simulink model "gnc"  (R2025b)
settings: Solver=ode2  StartTime=0.0  StopTime=inf  FixedStep=1/100  RelTol=1e-3
PreLoadFcn:
  | gnc_PreLoadFcn
undefined symbols (not defined in the file or in its folder): DiscIntNeverNeededParam, dspblkCoreblockFVToolHelper, gcbh
libraries: simulink_extras x7, simulink x5, eeGeneralControl x5
(part 2 of 4)

== system gnc/INDI/Monitor ==
  note: uint64 timestamp
      | float32[3] track_cmd
      | float32[3] track_m
      | float32[3] track_err
      | float32[3] gamma_dot_pid
      | float32[2] chi_dot_pd
      | float32[3] track_dot_cmd
      | float32[3] track_dot_m
      | float32[3] track_dot_err
      | float32[3] att_inc_cmd
      | float32[5] att_cmd
      | float32[5] att_m
      | float32[5] att_err
      | float32[5] att_dot_cmd
      | float32 delta_t
      | float32 t_m
      | float32 t_c
      | float32 chi_dot_cmd
      | float32 chi_dot_m
      | float32 chi_dot_err
      | float32 chi_ddot_cmd
      | float32[3] pqr_cmd
      | float32[3] pqr_m
      | float32[3] pqr_err
      | float32[3] pqr_dot_cmd
      | float32[3] pqr_dot_m
      | float32[3] pqr_dot_err
      | float32[3] delta_act
      | float32[3] act_m
      | float32[3] act_c
      | float32 nw_c
  note: float32[3] track_cmd
      | float32[3] track_m
      | float32[3] track_err
      | float32[3] gamma_dot_pid
      | float32[2] chi_dot_pd
      | float32[3] track_dot_cmd
      | float32[3] track_dot_m
      | float32[3] track_dot_err
      | float32[3] att_inc_cmd
  note: float32[5] att_cmd
      | float32[5] att_m
      | float32[5] att_err
      | float32[5] att_dot_cmd
  note: float32 delta_t
      | float32 t_m
      | float32 t_c
  note: float32 chi_dot_cmd
      | float32 chi_dot_m
      | float32 chi_dot_err
      | float32 chi_ddot_cmd
      | float32[3] pqr_cmd
      | float32[3] pqr_m
      | float32[3] pqr_err
      | float32[3] pqr_dot_cmd
      | float32[3] pqr_dot_m
      | float32[3] pqr_dot_err
      | float32[3] delta_act
      | float32[3] act_m
      | float32[3] act_c
      | float32 nw_c
  rte_moni : Inport  OutDataTypeStr=single  PortDimensions=32
  att_moni : Inport  Port=2  OutDataTypeStr=single  PortDimensions=20
  thr_moni : Inport  Port=3  OutDataTypeStr=single  PortDimensions=3
  path_moni : Inport  Port=4  OutDataTypeStr=single  PortDimensions=26
  Bus Creator1 : BusCreator  Inputs=31  OutDataTypeStr=Bus: indi_monitor_bus
      settings: InheritFromInputs=off
  Bus Selector1 : BusSelector  OutputSignals=signal1,signal2,signal3,signal4
  Bus Selector2 : BusSelector  OutputSignals=signal1.signal1,signal1.signal2,signal1.signal3,signal1.signal4,signal1.signal5,signal1.signal6,signal1.signal7,signal1.signal8,signal1.signal9,signal1.signal10,signal2.signal1,signal2.signal2,signal2.signal3,signal3
  Bus Selector3 : BusSelector  OutputSignals=signal1.signal1,signal1.signal2,signal1.signal3,signal1.signal4,signal1.signal5,signal1.signal6,signal1.signal7,signal1.signal8,att_inc_reciprocal
  Constant : Constant  OutDataTypeStr=boolean
  Demux4 : Demux  Outputs=3
  indi_monitor : Outport  OutDataTypeStr=Bus: indi_monitor_bus
  wires:
  thr_moni/1 -> Demux4/1
  Constant/1 -> Bus Creator1/1  "valid"
  Bus Creator1/1 -> indi_monitor/1
  Demux4/1 -> Bus Creator1/15
  Demux4/2 -> Bus Creator1/16
  Demux4/3 -> Bus Creator1/17
  Bus Selector2/1 -> Bus Creator1/18  "<signal1>"
  Bus Selector2/2 -> Bus Creator1/19  "<signal2>"
  Bus Selector2/3 -> Bus Creator1/20  "<signal3>"
  Bus Selector2/4 -> Bus Creator1/21  "<signal4>"
  Bus Selector2/5 -> Bus Creator1/22  "<signal5>"
  Bus Selector2/6 -> Bus Creator1/23  "<signal6>"
  Bus Selector2/8 -> Bus Creator1/25  "<signal8>"
  Bus Selector2/9 -> Bus Creator1/26  "<signal9>"
  Bus Selector2/10 -> Bus Creator1/27  "<signal10>"
  Bus Selector2/7 -> Bus Creator1/24  "<signal7>"
  Bus Selector2/14 -> Bus Creator1/31  "<signal3>"
  Bus Selector2/13 -> Bus Creator1/30  "<signal3>"
  Bus Selector2/11 -> Bus Creator1/28  "<signal1>"
  Bus Selector2/12 -> Bus Creator1/29  "<signal2>"
  Bus Selector3/1 -> Bus Creator1/2  "<signal1>"
  Bus Selector3/2 -> Bus Creator1/3  "<signal2>"
  Bus Selector3/3 -> Bus Creator1/4  "<signal3>"
  Bus Selector3/4 -> Bus Creator1/5  "<signal4>"
  Bus Selector3/5 -> Bus Creator1/6  "<signal5>"
  Bus Selector3/6 -> Bus Creator1/7  "<signal6>"
  Bus Selector3/7 -> Bus Creator1/8  "<signal7>"
  Bus Selector3/8 -> Bus Creator1/9  "<signal8>"
  Bus Selector1/1 -> Bus Creator1/11  "<signal1>"
  Bus Selector1/2 -> Bus Creator1/12  "<signal2>"
  Bus Selector1/3 -> Bus Creator1/13  "<signal3>"
  Bus Selector1/4 -> Bus Creator1/14  "<signal4>"
  path_moni/1 -> Bus Selector3/1
  att_moni/1 -> Bus Selector1/1
  rte_moni/1 -> Bus Selector2/1
  Bus Selector3/9 -> Bus Creator1/10  "<att_inc_reciprocal>"

== system gnc/INDI/Path ==
  note: [alpha,theta,beta,psi,mu]
  note: for attitude dynamics
  note: float32[3] track_cmd
      | float32[3] track_m
      | float32[3] track_err
      | float32[3] gamma_dot_pid
      | float32[2] chi_dot_pd
      | float32[3] track_dot_cmd
      | float32[3] track_dot_m
      | float32[3] track_dot_err
      | float32[3] att_inc_cmd
  gachiv_c : Inport  OutDataTypeStr=single  PortDimensions=3
  acc_k : Inport  Port=2
  Vk : Inport  Port=3  OutDataTypeStr=single  PortDimensions=1
  att_m : Inport  Port=4
  gachi_m : Inport  Port=5  OutDataTypeStr=single  PortDimensions=2
  track_deriv : Inport  Port=6
  params : Inport  Port=7  OutDataTypeStr=Bus: gnc_parameterBus
  q_dyn : Inport  Port=8
  Bus Creator : BusCreator  Inputs=2
  Incremental_inversion : Subsystem
  MATLAB Function : MATLAB Function  TreatAsAtomicUnit=on
  Mux1 : Mux  Inputs=2
  Mux3 : Mux  Inputs=2
  Pseudo-control : Subsystem
  Selector1 : Selector  InputPortWidth=5  IndexOptions=Index vector (dialog)  Indices=[1 3 5]  OutputSizes=1
  Selector2 : Selector  InputPortWidth=3  IndexOptions=Index vector (dialog)  Indices=3  OutputSizes=1
  Selector3 : Selector  InputPortWidth=5  IndexOptions=Index vector (dialog)  Indices=5  OutputSizes=1
  d/dt_gachiv_m : Outport  OutDataTypeStr=single  PortDimensions=3
  angles_c : Outport  Port=2  OutDataTypeStr=single  PortDimensions=5
  path_moni : Outport  Port=3
  thr_inc : Outport  Port=4  OutDataTypeStr=single  PortDimensions=1
  wires:
  Incremental_inversion/1(angles_c) -> angles_c/1
  att_m/1 -> Selector3/1, Selector1/1
  acc_k/1 -> MATLAB Function/1(acc_k)
  Pseudo-control/2(d/dt_gachiv_e) -> Incremental_inversion/1(d/dt_gachiv_e)
  Mux1/1 -> Incremental_inversion/3(gachiv_m), Pseudo-control/5(gachiv_m)
  gachi_m/1 -> Mux1/1
  Vk/1 -> Mux1/2, MATLAB Function/2(Vk)
  Selector1/1 -> Incremental_inversion/4(abmu_m)
  Selector3/1 -> Pseudo-control/4(phi_m)
  MATLAB Function/2(v_dot) -> Mux3/2
  Mux3/1 -> Pseudo-control/1(d/dt_gachiv_m), d/dt_gachiv_m/1
  params/1 -> Incremental_inversion/2(params), Pseudo-control/3(para)
  Incremental_inversion/2(inc_cmd) -> Bus Creator/2, Selector2/1
  q_dyn/1 -> Incremental_inversion/5(q_dyn)
  Pseudo-control/1(path_moni) -> Bus Creator/1
  track_deriv/1 -> Mux3/1
  Bus Creator/1 -> path_moni/1
  Selector2/1 -> thr_inc/1
  gachiv_c/1 -> Pseudo-control/2(gachiv_c)

== system gnc/INDI/Rates to surfaces&brakes ==
  note: float32 chi_dot_cmd
      | float32 chi_dot_m
      | float32 chi_dot_err
      | float32 chi_ddot_cmd
      | float32[3] pqr_cmd
      | float32[3] pqr_m
      | float32[3] pqr_err
      | float32[3] pqr_dot_cmd
      | float32[3] pqr_dot_m
      | float32[3] pqr_dot_err
      | float32[3] delta_act
      | float32[3] act_m
      | float32[3] act_c
      | float32 nw
  q_dyn : Inport
  rate_m : Inport  Port=2
  rate_ctrl : Inport  Port=3
  act_m : Inport  Port=4  OutDataTypeStr=single  PortDimensions=4
  params : Inport  Port=5  OutDataTypeStr=Bus: gnc_parameterBus
  inc_margins : Inport  Port=6  OutDataTypeStr=single  PortDimensions=[3,2]
  act_limits : Inport  Port=7
  imu_filter : Inport  Port=8
  Bus Creator : BusCreator  Inputs=3
  Constant : Constant  Value=0  OutDataTypeStr=single
  Demux : Demux  Outputs=3
  Diff and Filter IMU : Subsystem
      settings: PortSchema="{\"entries\":[{\"content\":{\"sides\":[{\"content\":{\"connectorIds\":[\"In1\",\"In2\",\"In3\"]},\"type\":\"ConnectorPlacement.EquallySpacedRectSide\",\"uuid\":\"595f2c85-6cd2-4ac4-94a6-147e3cdaf62c\"},{\"content\":{\"connectorIds\":[\"Out1\",\"Out2\"],\"side\":\"RIGHT\"},\"type\":\"ConnectorPlacement.EquallySpacedRectSide\",\"uuid\":\"fac480cf-7efe-4f97-8544-e0f640d96e89\"},{\"content\":{\"connectorIds\":[\"In4\"],\"side\":\"TOP\"},\"type\":\"ConnectorPlacement.EquallySpacedRectSide\",\"uuid\":\"db60b5ab-e407-476e-aa28-a63f2500fd6d\"}]},\"type\":\"ConnectorPlacement.EquallySpacedConnector\",\"uuid\":\"42848a63-649d-42c6-8a03-05f224ad5118\"}],\"packageUris\":[\"http://schema.mathworks.com/mf0/Connector/R2020b\"],\"version\":\"1.0\"}"
  Incremental_inversion : Subsystem
      settings: PortSchema="{\"entries\":[{\"content\":{\"sides\":[{\"content\":{\"connectorIds\":[\"In1\",\"In2\",\"In3\",\"In4\",\"In5\"]},\"type\":\"ConnectorPlacement.EquallySpacedRectSide\",\"uuid\":\"2477ed7f-2e4a-4d34-9191-aa6cd1598ace\"},{\"content\":{\"connectorIds\":[\"Out1\",\"Out2\",\"Out3\"],\"side\":\"RIGHT\"},\"type\":\"ConnectorPlacement.EquallySpacedRectSide\",\"uuid\":\"a67f6923-e928-4938-ab2a-8a1d443bfb45\"},{\"content\":{\"connectorIds\":[\"In6\"],\"side\":\"TOP\"},\"type\":\"ConnectorPlacement.EquallySpacedRectSide\",\"uuid\":\"ece43f97-e3a7-408a-af02-d9e4d3d20b00\"}]},\"type\":\"ConnectorPlacement.EquallySpacedConnector\",\"uuid\":\"8ca6f7dd-4284-4525-a7ce-c1aaa2c7f949\"}],\"packageUris\":[\"http://schema.mathworks.com/mf0/Connector/R2020b\"],\"version\":\"1.0\"}"
  Pseudo-control : Subsystem
      settings: PortSchema="{\"entries\":[{\"content\":{\"sides\":[{\"content\":{\"connectorIds\":[\"In1\",\"In2\",\"In3\"]},\"type\":\"ConnectorPlacement.EquallySpacedRectSide\",\"uuid\":\"2477ed7f-2e4a-4d34-9191-aa6cd1598ace\"},{\"content\":{\"connectorIds\":[\"Out1\",\"Out2\"],\"side\":\"RIGHT\"},\"type\":\"ConnectorPlacement.EquallySpacedRectSide\",\"uuid\":\"a67f6923-e928-4938-ab2a-8a1d443bfb45\"},{\"content\":{\"connectorIds\":[\"In4\"],\"side\":\"TOP\"},\"type\":\"ConnectorPlacement.EquallySpacedRectSide\",\"uuid\":\"ece43f97-e3a7-408a-af02-d9e4d3d20b00\"}]},\"type\":\"ConnectorPlacement.EquallySpacedConnector\",\"uuid\":\"8ca6f7dd-4284-4525-a7ce-c1aaa2c7f949\"}],\"packageUris\":[\"http://schema.mathworks.com/mf0/Connector/R2020b\"],\"version\":\"1.0\"}"
  Scope : Scope  NumInputPorts=3
      settings: ActiveDisplayYMinimum=-0.13287401574803148  ActiveDisplayYMaximum=0.13779527559055116  DataLoggingVariableName=ScopeData6
  control_surfaces : Outport  OutDataTypeStr=single  PortDimensions=3
  rte_moni : Outport  Port=2  OutDataTypeStr=single  PortDimensions=32
  inc_moni : Outport  Port=3
  wires:
  Incremental_inversion/1(act) -> control_surfaces/1, Demux/1
  Incremental_inversion/3(srfc_moni) -> Bus Creator/2
  Pseudo-control/2(rte_moni) -> Bus Creator/1
  params/1 -> Diff and Filter IMU/4(params), Pseudo-control/4(param), Incremental_inversion/6(params)
  rate_m/1 -> Diff and Filter IMU/3(rates), Pseudo-control/2(rate_m)
  Pseudo-control/1(d/dt_pqr_e) -> Incremental_inversion/5(d/dt_pqr_e)
  act_m/1 -> Diff and Filter IMU/2(act_m)
  Incremental_inversion/2(inc_moni) -> inc_moni/1
  Diff and Filter IMU/2(d/dt_pqr_m) -> Pseudo-control/1(pqr_dot_m)
  Bus Creator/1 -> rte_moni/1
  Demux/2 -> Scope/2  "ele_cmd"
  Demux/3 -> Scope/3  "rud_cmd"
  Demux/1 -> Scope/1  "ail_cmd"
  Diff and Filter IMU/1(act_del) -> Incremental_inversion/4(act_del)
  q_dyn/1 -> Incremental_inversion/3(q_dyn)
  inc_margins/1 -> Incremental_inversion/2(inc_margins)
  act_limits/1 -> Incremental_inversion/1(act_limits)
  imu_filter/1 -> Diff and Filter IMU/1(imu_filter)
  Constant/1 -> Bus Creator/3
  rate_ctrl/1 -> Pseudo-control/3(rte_c)

== system gnc/INDI/Thrust ==
  note: float32 delta_t
      | float32 t_m
      | float32 t_c
  note: Current thrust
      | lever in [-1,1]
  note: Incremental thrust
      | command in [-1,1]
  note: Total thrust
      | command in [0,1]
  thr_inc : Inport  OutDataTypeStr=single  PortDimensions=1
  act_m : Inport  Port=2  OutDataTypeStr=single  PortDimensions=4
  Bias : Bias  Bias=-1  SaturateOnIntegerOverflow=off
  Bias1 : Bias  Bias=0.5  SaturateOnIntegerOverflow=off
  Constant : Constant  OutDataTypeStr=single
  Constant1 : Constant  Value=-1  OutDataTypeStr=single
  Gain : Gain  Gain=2
  Gain1 : Gain  Gain=0.5
  Gain2 : Gain  Gain=0.5
  Limit_Increment : simulink/Discontinuities/Saturation Dynamic  OutMin=[]  OutMax=[]  OutDataTypeStr=Inherit: Same as second input  OutDataType=fixdt(1, 16)  OutScaling=2^-10  DoSatur=off
  Minus1 : Sum  Inputs=+-
  Minus2 : Sum  Inputs=+-
  Mux : Mux  Inputs=3
  Plus1 : Sum
  Scope : Scope  NumInputPorts=4
      settings: ActiveDisplayYMinimum=-2.22188  ActiveDisplayYMaximum=2.10921
  Selector1 : Selector  InputPortWidth=4  IndexOptions=Index vector (dialog)  Indices=4  OutputSizes=1
  thr_moni : Outport  OutDataTypeStr=single  PortDimensions=3
  thr : Outport  Port=2  OutDataTypeStr=single  PortDimensions=1
  inc_moni : Outport  Port=3
  wires:
  Mux/1 -> thr_moni/1
  Bias/1 -> Scope/1, Mux/2, Minus1/2, Minus2/2, Scope/3, Plus1/2
  Gain/1 -> Bias/1
  Limit_Increment/1 -> Plus1/1, Gain2/1, Scope/2, Mux/1  "thr_inc"
  act_m/1 -> Selector1/1
  Selector1/1 -> Gain/1
  Plus1/1 -> Gain1/1
  Gain1/1 -> Bias1/1
  Bias1/1 -> Scope/4, Mux/3, thr/1
  Gain2/1 -> inc_moni/1
  Constant/1 -> Minus1/1
  thr_inc/1 -> Limit_Increment/2
  Minus1/1 -> Limit_Increment/1
  Minus2/1 -> Limit_Increment/3
  Constant1/1 -> Minus2/1

== system gnc/Mixer/_bus_creator1 ==
  control : Inport  OutDataTypeStr=single  PortDimensions=8
  timestamp_sample : Inport  Port=2  OutDataTypeStr=double  PortDimensions=1
  Bus Creator : BusCreator  Inputs=20  OutDataTypeStr=Bus:actuator_controls_0_bus
      settings: InheritFromInputs=off
  GROUP_INDEX_ATTITUDE : Constant  Value=0  OutDataTypeStr=uint8
  GROUP_INDEX_ATTITUDE_ALTERNATE : Constant  OutDataTypeStr=uint8
  GROUP_INDEX_GIMBAL : Constant  Value=2  OutDataTypeStr=uint8
  GROUP_INDEX_MANUAL_PASSTHROUGH : Constant  Value=3  OutDataTypeStr=uint8
  GROUP_INDEX_PAYLOAD : Constant  Value=6  OutDataTypeStr=uint8
  INDEX_AIRBRAKES : Constant  Value=6  OutDataTypeStr=uint8
  INDEX_CAMERA_ZOOM : Constant  Value=4  OutDataTypeStr=uint8
  INDEX_FLAPS : Constant  Value=4  OutDataTypeStr=uint8
  INDEX_GIMBAL_SHUTTER : Constant  Value=3  OutDataTypeStr=uint8
  INDEX_LANDING_GEAR : Constant  Value=7  OutDataTypeStr=uint8
  INDEX_PITCH : Constant  OutDataTypeStr=uint8
  INDEX_ROLL : Constant  Value=0  OutDataTypeStr=uint8
  INDEX_SPOILERS : Constant  Value=5  OutDataTypeStr=uint8
  INDEX_THROTTLE : Constant  Value=3  OutDataTypeStr=uint8
  INDEX_YAW : Constant  Value=2  OutDataTypeStr=uint8
  NUM_ACTUATOR_CONTROLS : Constant  Value=8  OutDataTypeStr=uint8
  NUM_ACTUATOR_CONTROL_GROUPS : Constant  Value=4  OutDataTypeStr=uint8
  is_valid : Constant  Value=true  OutDataTypeStr=boolean
  actuator_controls : Outport  OutDataTypeStr=Bus:actuator_controls_0_bus  VectorParamsAs1DForOutWhenUnconnected=off
  wires:
  Bus Creator/1 -> actuator_controls/1
  control/1 -> Bus Creator/20
  timestamp_sample/1 -> Bus Creator/19
  GROUP_INDEX_ATTITUDE_ALTERNATE/1 -> Bus Creator/15
  GROUP_INDEX_ATTITUDE/1 -> Bus Creator/14
  INDEX_LANDING_GEAR/1 -> Bus Creator/11
  INDEX_AIRBRAKES/1 -> Bus Creator/10
  INDEX_SPOILERS/1 -> Bus Creator/9
  INDEX_FLAPS/1 -> Bus Creator/8
  INDEX_THROTTLE/1 -> Bus Creator/7
  INDEX_YAW/1 -> Bus Creator/6
  INDEX_PITCH/1 -> Bus Creator/5
  INDEX_ROLL/1 -> Bus Creator/4
  NUM_ACTUATOR_CONTROL_GROUPS/1 -> Bus Creator/3
  NUM_ACTUATOR_CONTROLS/1 -> Bus Creator/2
  is_valid/1 -> Bus Creator/1
  INDEX_GIMBAL_SHUTTER/1 -> Bus Creator/12
  INDEX_CAMERA_ZOOM/1 -> Bus Creator/13
  GROUP_INDEX_GIMBAL/1 -> Bus Creator/16
  GROUP_INDEX_MANUAL_PASSTHROUGH/1 -> Bus Creator/17
  GROUP_INDEX_PAYLOAD/1 -> Bus Creator/18

== system gnc/Mixer/_bus_creator2 ==
  control : Inport  OutDataTypeStr=single  PortDimensions=8
  timestamp_sample : Inport  Port=2  OutDataTypeStr=double  PortDimensions=1
  Bus Creator : BusCreator  Inputs=20  OutDataTypeStr=Bus:actuator_controls_0_bus
      settings: InheritFromInputs=off
  GROUP_INDEX_ATTITUDE : Constant  Value=0  OutDataTypeStr=uint8
  GROUP_INDEX_ATTITUDE_ALTERNATE : Constant  OutDataTypeStr=uint8
  GROUP_INDEX_GIMBAL : Constant  Value=2  OutDataTypeStr=uint8
  GROUP_INDEX_MANUAL_PASSTHROUGH : Constant  Value=3  OutDataTypeStr=uint8
  GROUP_INDEX_PAYLOAD : Constant  Value=6  OutDataTypeStr=uint8
  INDEX_AIRBRAKES : Constant  Value=6  OutDataTypeStr=uint8
  INDEX_CAMERA_ZOOM : Constant  Value=4  OutDataTypeStr=uint8
  INDEX_FLAPS : Constant  Value=4  OutDataTypeStr=uint8
  INDEX_GIMBAL_SHUTTER : Constant  Value=3  OutDataTypeStr=uint8
  INDEX_LANDING_GEAR : Constant  Value=7  OutDataTypeStr=uint8
  INDEX_PITCH : Constant  OutDataTypeStr=uint8
  INDEX_ROLL : Constant  Value=0  OutDataTypeStr=uint8
  INDEX_SPOILERS : Constant  Value=5  OutDataTypeStr=uint8
  INDEX_THROTTLE : Constant  Value=3  OutDataTypeStr=uint8
  INDEX_YAW : Constant  Value=2  OutDataTypeStr=uint8
  NUM_ACTUATOR_CONTROLS : Constant  Value=8  OutDataTypeStr=uint8
  NUM_ACTUATOR_CONTROL_GROUPS : Constant  Value=4  OutDataTypeStr=uint8
  is_valid : Constant  Value=true  OutDataTypeStr=boolean
  actuator_controls : Outport  OutDataTypeStr=Bus:actuator_controls_1_bus  VectorParamsAs1DForOutWhenUnconnected=off
  wires:
  INDEX_ROLL/1 -> Bus Creator/4
  INDEX_SPOILERS/1 -> Bus Creator/9
  is_valid/1 -> Bus Creator/1
  INDEX_CAMERA_ZOOM/1 -> Bus Creator/13
  control/1 -> Bus Creator/20
  GROUP_INDEX_ATTITUDE_ALTERNATE/1 -> Bus Creator/15
  GROUP_INDEX_GIMBAL/1 -> Bus Creator/16
  INDEX_GIMBAL_SHUTTER/1 -> Bus Creator/12
  INDEX_THROTTLE/1 -> Bus Creator/7
  GROUP_INDEX_ATTITUDE/1 -> Bus Creator/14
  Bus Creator/1 -> actuator_controls/1
  INDEX_PITCH/1 -> Bus Creator/5
  GROUP_INDEX_MANUAL_PASSTHROUGH/1 -> Bus Creator/17
  INDEX_FLAPS/1 -> Bus Creator/8
  INDEX_AIRBRAKES/1 -> Bus Creator/10
  NUM_ACTUATOR_CONTROLS/1 -> Bus Creator/2
  GROUP_INDEX_PAYLOAD/1 -> Bus Creator/18
  timestamp_sample/1 -> Bus Creator/19
  INDEX_YAW/1 -> Bus Creator/6
  NUM_ACTUATOR_CONTROL_GROUPS/1 -> Bus Creator/3
  INDEX_LANDING_GEAR/1 -> Bus Creator/11

== system gnc/Modal/Subsystem2 ==
  note: [ Eta    ]
      | [ Delta ]
  mode : Inport
  dx : Inport  Port=2
  u0 : Inport  Port=3
  u : Inport  Port=4
  param : Inport  Port=5
  Constant : Constant  Value=0
  Delay : Delay  DelayLength=1
  Demux : Demux  Outputs=2
  Demux1 : Demux  Outputs=2
  Demux2 : Demux  Outputs=2
  Detect Change : simulink/Logic and Bit Operations/Detect Change  vinit=0  OutDataTypeStr=boolean
  Discrete-Time Integrator : DiscreteIntegrator  ExternalReset=sampled level  InitialConditionSource=external  SampleTime=-1  ShowStatePort=on  ICPrevOutput=DiscIntNeverNeededParam  ICPrevScaledInput=DiscIntNeverNeededParam
  Discrete-Time Integrator1 : DiscreteIntegrator  ExternalReset=sampled level  InitialConditionSource=external  SampleTime=-1  ShowStatePort=on  ICPrevOutput=DiscIntNeverNeededParam  ICPrevScaledInput=DiscIntNeverNeededParam
  MATLAB Function : MATLAB Function  TreatAsAtomicUnit=on
  MATLAB Function1 : MATLAB Function  TreatAsAtomicUnit=on
  Mux : Mux  Inputs=2
  Scope : Scope  NumInputPorts=3
      settings: ActiveDisplayYMinimum=-0.37499999999999989  ActiveDisplayYMaximum=3.375  DataLoggingVariableName=ScopeData32
  Scope1 : Scope  NumInputPorts=4
      settings: ActiveDisplayYMinimum=-7.2987606078386307  ActiveDisplayYMaximum=2.4926107674837112  DataLoggingVariableName=ScopeData33
  Scope2 : Scope  NumInputPorts=4
      settings: DataLoggingVariableName=ScopeData34
  Selector4 : Selector  InputPortWidth=4  IndexOptions=Index vector (dialog)  Indices=[2 4]  OutputSizes=1
  Switch : Switch  Criteria=u2 > Threshold  SaturateOnIntegerOverflow=off  InputSameDT=off
  x : Outport  VectorParamsAs1DForOutWhenUnconnected=off
  wires:
  Constant/1 -> Switch/3
  Detect Change/1 -> Scope/2, Switch/1  "external trigger"
  Delay/1 -> Switch/2
  Selector4/1 -> Demux1/1
  Discrete-Time Integrator1/1 -> Mux/2, Scope2/4  "x"
  Mux/1 -> x/1
  Discrete-Time Integrator/1 -> Mux/1, Scope1/4
  Demux1/1 -> MATLAB Function/3(u0)
  Demux/2 -> MATLAB Function1/4(u)  "u"
  Demux/1 -> MATLAB Function/4(u)
  Demux1/2 -> MATLAB Function1/3(u0)
  Demux2/2 -> Scope2/1, Discrete-Time Integrator1/1
  Demux2/1 -> Scope1/1, Discrete-Time Integrator/1
  Discrete-Time Integrator1/State -> MATLAB Function1/1(x)
  dx/1 -> Demux2/1
  u0/1 -> Selector4/1
  MATLAB Function1/1(trigger) -> Scope2/3, Discrete-Time Integrator1/2  "general trigger"
  MATLAB Function1/2(x0) -> Scope2/2, Discrete-Time Integrator1/3
  Switch/1 -> MATLAB Function1/2(external), MATLAB Function/2(external), Scope/3  "external trigger"
  Discrete-Time Integrator/State -> MATLAB Function/1(x)
  mode/1 -> Delay/1, Scope/1, Detect Change/1
  MATLAB Function/2(x0) -> Scope1/2, Discrete-Time Integrator/3
  MATLAB Function/1(trigger) -> Scope1/3, Discrete-Time Integrator/2
  u/1 -> Demux/1
  param/1 -> MATLAB Function/5(param), MATLAB Function1/5(param)

== system gnc/Subsystem2/Actuator_Model ==
  rc_channel : Inport
  main_axes : Inport  Port=2  OutDataTypeStr=Bus: main_ctrl_axes_bus
  act_lims : Inport  Port=3
  Actuator Model : Subsystem
  Subsystem1 : Subsystem
  act_m : Outport
  rc_mode : Outport  Port=2  OutDataTypeStr=uint8
  rc_trim : Outport  Port=3  PortDimensions=4
  wires:
  Subsystem1/1(rc_mode) -> rc_mode/1
  act_lims/1 -> Actuator Model/4(act_lims)
  main_axes/1 -> Actuator Model/3(AP_controls)
  Actuator Model/1(Delayed) -> act_m/1
  Subsystem1/2(RC_controls) -> Actuator Model/1(RC_controls), rc_trim/1
  Subsystem1/3(Safety_Switch) -> Actuator Model/2(Safety_Switch)
  rc_channel/1 -> Subsystem1/1(RC_channels)

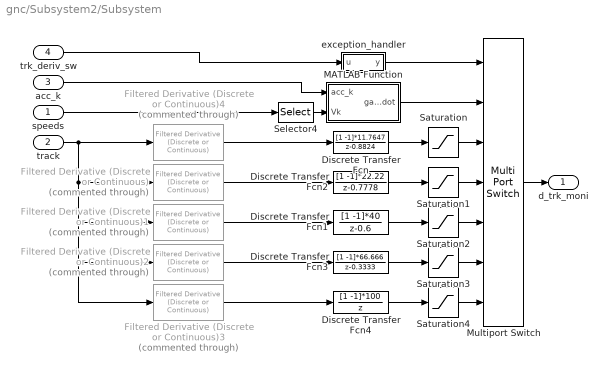
== system gnc/Subsystem2/Subsystem ==
  speeds : Inport
  track : Inport  Port=2
  acc_k : Inport  Port=3
  trk_deriv_sw : Inport  Port=4
  Discrete Transfer Fcn : DiscreteTransferFcn  LoadFcn=dspblkCoreblockFVToolHelper(gcbh,'load');  Numerator=[1 -1]*11.7647  Denominator=[1 -0.8824]
      settings: CopyFcn=dspblkCoreblockFVToolHelper(gcbh,'copy');  DeleteFcn=dspblkCoreblockFVToolHelper(gcbh,'close');  ModelCloseFcn=dspblkCoreblockFVToolHelper(gcbh,'close');  PreSaveFcn=dspblkCoreblockFVToolHelper(gcbh,'presave');  PostSaveFcn=dspblkCoreblockFVToolHelper(gcbh,'postsave');  CloseFcn=dspblkCoreblockFVToolHelper(gcbh,'close');
  Discrete Transfer Fcn1 : DiscreteTransferFcn  LoadFcn=dspblkCoreblockFVToolHelper(gcbh,'load');  Numerator=[1 -1]*40  Denominator=[1 -0.6]
      settings: CopyFcn=dspblkCoreblockFVToolHelper(gcbh,'copy');  DeleteFcn=dspblkCoreblockFVToolHelper(gcbh,'close');  ModelCloseFcn=dspblkCoreblockFVToolHelper(gcbh,'close');  PreSaveFcn=dspblkCoreblockFVToolHelper(gcbh,'presave');  PostSaveFcn=dspblkCoreblockFVToolHelper(gcbh,'postsave');  CloseFcn=dspblkCoreblockFVToolHelper(gcbh,'close');
  Discrete Transfer Fcn2 : DiscreteTransferFcn  LoadFcn=dspblkCoreblockFVToolHelper(gcbh,'load');  Numerator=[1 -1]*22.22  Denominator=[1 -0.7778]
      settings: CopyFcn=dspblkCoreblockFVToolHelper(gcbh,'copy');  DeleteFcn=dspblkCoreblockFVToolHelper(gcbh,'close');  ModelCloseFcn=dspblkCoreblockFVToolHelper(gcbh,'close');  PreSaveFcn=dspblkCoreblockFVToolHelper(gcbh,'presave');  PostSaveFcn=dspblkCoreblockFVToolHelper(gcbh,'postsave');  CloseFcn=dspblkCoreblockFVToolHelper(gcbh,'close');
  Discrete Transfer Fcn3 : DiscreteTransferFcn  LoadFcn=dspblkCoreblockFVToolHelper(gcbh,'load');  Numerator=[1 -1]*66.666  Denominator=[1 -0.3333]
      settings: CopyFcn=dspblkCoreblockFVToolHelper(gcbh,'copy');  DeleteFcn=dspblkCoreblockFVToolHelper(gcbh,'close');  ModelCloseFcn=dspblkCoreblockFVToolHelper(gcbh,'close');  PreSaveFcn=dspblkCoreblockFVToolHelper(gcbh,'presave');  PostSaveFcn=dspblkCoreblockFVToolHelper(gcbh,'postsave');  CloseFcn=dspblkCoreblockFVToolHelper(gcbh,'close');
  Discrete Transfer Fcn4 : DiscreteTransferFcn  LoadFcn=dspblkCoreblockFVToolHelper(gcbh,'load');  Numerator=[1 -1]*100  Denominator=[1 0]
      settings: CopyFcn=dspblkCoreblockFVToolHelper(gcbh,'copy');  DeleteFcn=dspblkCoreblockFVToolHelper(gcbh,'close');  ModelCloseFcn=dspblkCoreblockFVToolHelper(gcbh,'close');  PreSaveFcn=dspblkCoreblockFVToolHelper(gcbh,'presave');  PostSaveFcn=dspblkCoreblockFVToolHelper(gcbh,'postsave');  CloseFcn=dspblkCoreblockFVToolHelper(gcbh,'close');
  Filtered Derivative (Discrete or Continuous) : eeGeneralControl/Filtered Derivative (Discrete or Continuous)  Commented=through  K=1  T=0.04  B=inf  A=-inf  minRatio=10  init_option=Inherited from block input  x0=0  Ts=-1
      settings: LibrarySourceBlock=|
      | ee_sl_lib/General Control/Filtered Derivative
      | (Discrete or Continuous)
  Filtered Derivative (Discrete or Continuous)1 : eeGeneralControl/Filtered Derivative (Discrete or Continuous)  Commented=through  K=1  T=0.02  B=inf  A=-inf  minRatio=10  init_option=Inherited from block input  x0=0  Ts=-1
      settings: LibrarySourceBlock=|
      | ee_sl_lib/General Control/Filtered Derivative
      | (Discrete or Continuous)
  Filtered Derivative (Discrete or Continuous)2 : eeGeneralControl/Filtered Derivative (Discrete or Continuous)  Commented=through  K=1  T=0.01  B=inf  A=-inf  minRatio=10  init_option=Inherited from block input  x0=0  Ts=-1
      settings: LibrarySourceBlock=|
      | ee_sl_lib/General Control/Filtered Derivative
      | (Discrete or Continuous)
  Filtered Derivative (Discrete or Continuous)3 : eeGeneralControl/Filtered Derivative (Discrete or Continuous)  Commented=through  K=1  T=0.005  B=inf  A=-inf  minRatio=10  init_option=Inherited from block input  x0=0  Ts=-1
      settings: LibrarySourceBlock=|
      | ee_sl_lib/General Control/Filtered Derivative
      | (Discrete or Continuous)
  Filtered Derivative (Discrete or Continuous)4 : eeGeneralControl/Filtered Derivative (Discrete or Continuous)  Commented=through  K=1  T=0.08  B=inf  A=-inf  minRatio=10  init_option=Inherited from block input  x0=0  Ts=-1
      settings: LibrarySourceBlock=|
      | ee_sl_lib/General Control/Filtered Derivative
      | (Discrete or Continuous)
  MATLAB Function : MATLAB Function  TreatAsAtomicUnit=on
  Multiport Switch : MultiPortSwitch  Inputs=6  SaturateOnIntegerOverflow=off  InputSameDT=off
  Saturation{,1..4} (5 alike) : Saturate  UpperLimit=pi  LowerLimit=-pi
  Selector4 : Selector  InputPortWidth=2  IndexOptions=Index vector (dialog)  Indices=1  OutputSizes=1
  exception_handler : MATLAB Function  TreatAsAtomicUnit=on
  d_trk_moni : Outport  PortDimensions=2
  wires:
  exception_handler/1(y) -> Multiport Switch/1
  speeds/1 -> Selector4/1
  Saturation/1 -> Multiport Switch/3
  Discrete Transfer Fcn1/1 -> Saturation2/1
  MATLAB Function/1(gachi_dot) -> Multiport Switch/2
  Saturation1/1 -> Multiport Switch/4
  Filtered Derivative (Discrete or Continuous)4/1 -> Discrete Transfer Fcn/1
  acc_k/1 -> MATLAB Function/1(acc_k)
  Filtered Derivative (Discrete or Continuous)/1 -> Discrete Transfer Fcn2/1
  track/1 -> Filtered Derivative (Discrete or Continuous)4/1, Filtered Derivative (Discrete or Continuous)/1, Filtered Derivative (Discrete or Continuous)1/1, Filtered Derivative (Discrete or Continuous)2/1, Filtered Derivative (Discrete or Continuous)3/1
  Filtered Derivative (Discrete or Continuous)1/1 -> Discrete Transfer Fcn1/1
  Discrete Transfer Fcn4/1 -> Saturation4/1
  Saturation4/1 -> Multiport Switch/7
  Discrete Transfer Fcn2/1 -> Saturation1/1
  Discrete Transfer Fcn/1 -> Saturation/1
  Selector4/1 -> MATLAB Function/2(Vk)
  Discrete Transfer Fcn3/1 -> Saturation3/1
  Filtered Derivative (Discrete or Continuous)2/1 -> Discrete Transfer Fcn3/1
  Saturation2/1 -> Multiport Switch/5
  Filtered Derivative (Discrete or Continuous)3/1 -> Discrete Transfer Fcn4/1
  Saturation3/1 -> Multiport Switch/6
  trk_deriv_sw/1 -> exception_handler/1(u)
  Multiport Switch/1 -> d_trk_moni/1

== system gnc/Subsystem2/Subsystem1 ==
  acc_g_vlp : Inport
  acc_g_filt : Inport  Port=2
  acc_k : Inport  Port=3
  Bus Creator1 : BusCreator  Inputs=4  OutDataTypeStr=Bus: accel_monitor_bus
      settings: InheritFromInputs=off
  Scope : Scope  NumInputPorts=3
      settings: ActiveDisplayYMinimum=-9.3330631852149963  ActiveDisplayYMaximum=8.4078307747840881  DataLoggingVariableName=ScopeData36
  timestamp : Constant  Value=0  OutDataTypeStr=boolean
  acc_moni : Outport  OutDataTypeStr=Bus: accel_monitor_bus
  wires:
  Bus Creator1/1 -> acc_moni/1
  timestamp/1 -> Bus Creator1/1
  acc_g_vlp/1 -> Scope/1, Bus Creator1/2
  acc_g_filt/1 -> Scope/2, Bus Creator1/3
  acc_k/1 -> Scope/3, Bus Creator1/4

== system gnc/Subsystem2/Subsystem2 ==
  track_deriv : Inport  OutDataTypeStr=Bus: track_deriv_monitor_bus
  trk_deriv_sw : Inport  Port=2
  Bus Selector : BusSelector  OutputSignals=gamma_dot_acc,chi_dot_acc,gamma_dot_der_008,chi_dot_der_008,gamma_dot_der_004,chi_dot_der_004,gamma_dot_der_002,chi_dot_der_002,gamma_dot_der_001,chi_dot_der_001,gamma_dot_der_0005,chi_dot_der_0005
  Multiport Switch : MultiPortSwitch  Inputs=6  SaturateOnIntegerOverflow=off  InputSameDT=off
  Mux{2,4..8} (6 alike) : Mux  Inputs=2
  exception_handler : MATLAB Function  TreatAsAtomicUnit=on
  trk_deriv : Outport  PortDimensions=2
  wires:
  exception_handler/1(y) -> Multiport Switch/1
  Bus Selector/2 -> Mux7/2  "<chi_dot_acc>"
  Mux4/1 -> Multiport Switch/7
  Bus Selector/6 -> Mux5/2  "<chi_dot_der_004>"
  Multiport Switch/1 -> trk_deriv/1
  Bus Selector/4 -> Mux8/2  "<chi_dot_der_008>"
  track_deriv/1 -> Bus Selector/1
  Bus Selector/1 -> Mux7/1  "<gamma_dot_acc>"
  Bus Selector/5 -> Mux5/1  "<gamma_dot_der_004>"
  Bus Selector/12 -> Mux4/2  "<chi_dot_der_0005>"
  trk_deriv_sw/1 -> exception_handler/1(u)
  Mux7/1 -> Multiport Switch/2
  Bus Selector/3 -> Mux8/1  "<gamma_dot_der_008>"
  Bus Selector/11 -> Mux4/1  "<gamma_dot_der_0005>"
  Bus Selector/10 -> Mux2/2  "<chi_dot_der_001>"
  Mux8/1 -> Multiport Switch/3
  Bus Selector/7 -> Mux6/1  "<gamma_dot_der_002>"
  Mux5/1 -> Multiport Switch/4
  Bus Selector/9 -> Mux2/1  "<gamma_dot_der_001>"
  Bus Selector/8 -> Mux6/2  "<chi_dot_der_002>"
  Mux2/1 -> Multiport Switch/6
  Mux6/1 -> Multiport Switch/5

== system gnc/Subsystem2/Subsystem3 ==
  RC_trim : Inport  OutDataTypeStr=Bus: rc_trim_bus
  Bus Selector2 : BusSelector  OutputSignals=aileron,elevator,rudder,thrust
  Mux2 : Mux
  rc_controls : Outport  PortDimensions=4
  wires:
  Bus Selector2/2 -> Mux2/2  "<elevator>"
  Bus Selector2/3 -> Mux2/3  "<rudder>"
  Bus Selector2/1 -> Mux2/1  "<aileron>"
  Bus Selector2/4 -> Mux2/4  "<thrust>"
  RC_trim/1 -> Bus Selector2/1
  Mux2/1 -> rc_controls/1

== system gnc/INDI/Attitude/Nonlinear_inversion ==
  d/dt_att_c : Inport
  param : Inport  Port=2  OutDataTypeStr=Bus: gnc_parameterBus
  att_m : Inport  Port=3
  modes : Inport  Port=4
  d/dt_gachiv_m : Inport  Port=5  OutDataTypeStr=single  PortDimensions=3
  path_m : Inport  Port=6
  Limit_command : MATLAB Function  TreatAsAtomicUnit=on
  Rate_Command_Generator : MATLAB Function  TreatAsAtomicUnit=on
  Selector : Selector  InputPortWidth=2  IndexOptions=Index vector (dialog)  Indices=1  OutputSizes=1
  rates_ltd : Outport
  wires:
  path_m/1 -> Selector/1
  Selector/1 -> Rate_Command_Generator/3(gamma_m)
  att_m/1 -> Rate_Command_Generator/5(att_m)
  Rate_Command_Generator/1(pqr_cmd) -> Limit_command/2(pqr_c)
  param/1 -> Limit_command/1(param)
  d/dt_att_c/1 -> Rate_Command_Generator/1(att_dot_cmd)
  d/dt_gachiv_m/1 -> Rate_Command_Generator/2(gachiv_dot_m)
  Limit_command/1(rates_ltd) -> rates_ltd/1
  modes/1 -> Rate_Command_Generator/4(modes)

== system gnc/INDI/Attitude/Pseudo-control ==
  note: float32[5] att_cmd
      | float32[5] att_m
      | float32[5] att_err
      | float32[5] att_dot_cmd
  note: Control error
  note: Control gain
  att_c : Inport  OutDataTypeStr=single  PortDimensions=5
  roll_lim : Inport  Port=2  OutDataTypeStr=single  PortDimensions=1
  att_m : Inport  Port=3  OutDataTypeStr=single  PortDimensions=5
  param : Inport  Port=4  OutDataTypeStr=Bus: gnc_parameterBus
  Bus Creator : BusCreator  Inputs=4
  Bus Selector : BusSelector  OutputSignals=indi.K_ATT_ALPHA,indi.K_ATT_THETA,indi.K_ATT_BETA,indi.K_ATT_PSI,indi.K_ATT_PHI
  Gain{,2..4,11..12} (6 alike) : Gain  Gain=180/pi*ones(5,1)
  Limit_angles : MATLAB Function  TreatAsAtomicUnit=on
  Mux1 : Mux  Inputs=5
  Product2 : Product
  Scope : Scope  NumInputPorts=2
      settings: ActiveDisplayYMinimum=-1206.3319816589355  ActiveDisplayYMaximum=675.23673629760742  DataLoggingVariableName=ScopeData3
  Scope1 : Scope  NumInputPorts=4
      settings: ActiveDisplayYMinimum=-1  ActiveDisplayYMaximum=1
  Sum1 : Sum  Inputs=-+|
  att_moni : Outport  OutDataTypeStr=single  PortDimensions=20
  d/dt_att_c : Outport  Port=2  OutDataTypeStr=single  PortDimensions=5
  wires:
  Mux1/1 -> Product2/1
  att_c/1 -> Gain3/1, Limit_angles/2(att_c)
  Product2/1 -> Gain/1, d/dt_att_c/1
  Bus Selector/3 -> Mux1/3  "<K_ATT_BETA>"
  Bus Selector/1 -> Mux1/1  "<K_ATT_ALPHA>"
  Bus Selector/4 -> Mux1/4  "<K_ATT_PSI>"
  Bus Selector/2 -> Mux1/2  "<K_ATT_THETA>"
  Bus Selector/5 -> Mux1/5  "<K_ATT_PHI>"
  Limit_angles/1(ltd) -> Sum1/2, Gain2/1
  Gain/1 -> Bus Creator/4, Scope/1
  Gain2/1 -> Scope1/2
  Gain3/1 -> Bus Creator/1, Scope1/3
  Gain4/1 -> Bus Creator/2, Scope1/4
  Bus Creator/1 -> att_moni/1
  Sum1/1 -> Gain12/1, Gain11/1, Product2/2
  att_m/1 -> Gain4/1, Sum1/1
  Gain12/1 -> Bus Creator/3, Scope/2
  Gain11/1 -> Scope1/1
  roll_lim/1 -> Limit_angles/3(roll_limit)
  param/1 -> Limit_angles/1(params), Bus Selector/1

== system gnc/INDI/Path/Incremental_inversion ==
  note: [alpha,theta,beta,psi,mu]
  d/dt_gachiv_e : Inport
  params : Inport  Port=2  OutDataTypeStr=Bus: gnc_parameterBus
  gachiv_m : Inport  Port=3  OutDataTypeStr=single  PortDimensions=3
  abmu_m : Inport  Port=4
  q_dyn : Inport  Port=5
  Attitude_Command_Generator : MATLAB Function  TreatAsAtomicUnit=on
  Constant : Constant  Value=0  OutDataTypeStr=single
  Demux1 : Demux  Outputs=3
  Demux2 : Demux  Outputs=2
  Demux5 : Demux  Outputs=3
  Gain10 : Gain  Gain=180/pi
  Gain9 : Gain  Gain=[180/pi,180/pi,1]
  Minus2 : Sum  Inputs=+-
  Mux : Mux  Inputs=2
  Mux1 : Mux  Inputs=2
  Mux12 : Mux  Inputs=5
  Plus : Sum
  Scope2 : Scope  NumInputPorts=3
      settings: ActiveDisplayYMinimum=-0.066928728080398514  ActiveDisplayYMaximum=0.84679823333079618
  Scope6 : Scope  NumInputPorts=2
      settings: ActiveDisplayYMinimum=-54.584307008348048  ActiveDisplayYMaximum=22.013184027047203  DataLoggingVariableName=ScopeData16
  Selector : Selector  InputPortWidth=3  IndexOptions=Index vector (dialog)  Indices=[1,3]  OutputSizes=1
  angles_c : Outport  OutDataTypeStr=single  PortDimensions=5
  inc_cmd : Outport  Port=2  OutDataTypeStr=single  PortDimensions=3
  wires:
  q_dyn/1 -> Attitude_Command_Generator/5(q_dyn)
  Gain10/1 -> Scope6/2
  Gain9/1 -> Scope6/1
  Attitude_Command_Generator/1(att_inc_reciprocal) -> inc_cmd/1, Demux5/1, Scope2/3, Minus2/2
  Minus2/1 -> Scope2/1
  Attitude_Command_Generator/2(att_inc_inversion) -> Minus2/1, Scope2/2
  Selector/1 -> Attitude_Command_Generator/4(gav_m)
  gachiv_m/1 -> Selector/1
  d/dt_gachiv_e/1 -> Gain9/1, Attitude_Command_Generator/1(gachiv_dot_e)
  abmu_m/1 -> Demux1/1, Attitude_Command_Generator/2(abmu_m)
  Mux12/1 -> Gain10/1, angles_c/1
  params/1 -> Attitude_Command_Generator/3(params)
  Constant/1 -> Mux12/2, Mux12/4, Mux12/3
  Demux2/2 -> Mux12/5
  Demux5/2 -> Mux/2
  Demux5/1 -> Mux/1
  Mux/1 -> Plus/2
  Mux1/1 -> Plus/1
  Demux1/1 -> Mux1/1
  Demux1/3 -> Mux1/2
  Demux2/1 -> Mux12/1
  Plus/1 -> Demux2/1

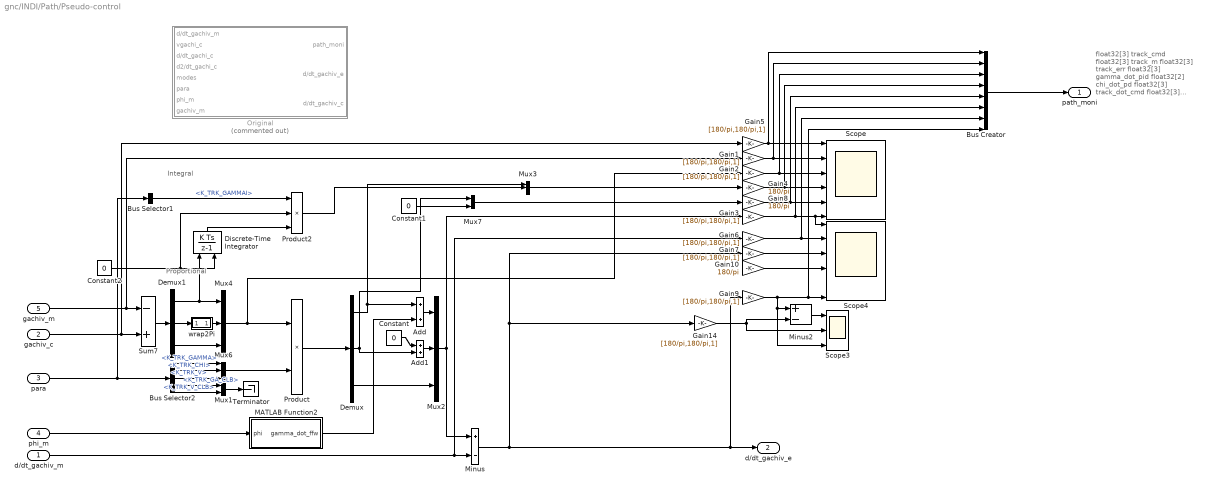
== system gnc/INDI/Path/Pseudo-control ==
  note: Proportional
  note: Integral
  note: float32[3] track_cmd
      | float32[3] track_m
      | float32[3] track_err
      | float32[3] gamma_dot_pid
      | float32[2] chi_dot_pd
      | float32[3] track_dot_cmd
      | float32[3] track_dot_m
      | float32[3] track_dot_err
  d/dt_gachiv_m : Inport  PortDimensions=3
  gachiv_c : Inport  Port=2
  para : Inport  Port=3  OutDataTypeStr=Bus: gnc_parameterBus
  phi_m : Inport  Port=4
  gachiv_m : Inport  Port=5  PortDimensions=3
  Add : Sum
  Add1 : Sum
  Bus Creator : BusCreator  Inputs=8
  Bus Selector1 : BusSelector  OutputSignals=indi.K_TRK_GAMMAI
  Bus Selector2 : BusSelector  OutputSignals=indi.K_TRK_GAMMA,indi.K_TRK_CHI,indi.K_TRK_V,indi.K_TRK_GA_CLB,indi.K_TRK_V_CLB
  Constant : Constant  Value=0  OutDataTypeStr=single
  Constant1 : Constant  Value=0  OutDataTypeStr=single
  Constant2 : Constant  Value=0  OutDataTypeStr=boolean
  Demux : Demux  Outputs=3
  Demux1 : Demux  Outputs=3
  Discrete-Time Integrator : DiscreteIntegrator  ExternalReset=rising  SampleTime=-1  LimitOutput=on  UpperSaturationLimit=1  LowerSaturationLimit=-1  ICPrevOutput=DiscIntNeverNeededParam  ICPrevScaledInput=DiscIntNeverNeededParam
  Gain{1..3,5..7,9,14} (8 alike) : Gain  Gain=[180/pi,180/pi,1]
  Gain10 : Gain  Gain=180/pi
  Gain4 : Gain  Gain=180/pi
  Gain8 : Gain  Gain=180/pi
  MATLAB Function2 : MATLAB Function  TreatAsAtomicUnit=on
  Minus : Sum  Inputs=+-
  Minus2 : Sum  Inputs=+-
  Mux1 : Mux  Inputs=2
  Mux{2..4,6} (4 alike) : Mux  Inputs=3
  Mux7 : Mux  Inputs=2
  Original : Subsystem  Commented=on
  Product : Product
  Product2 : Product  Inputs=3
  Scope : Scope  NumInputPorts=6
      settings: ActiveDisplayYMinimum=-158.91892623901367  ActiveDisplayYMaximum=214.35160446166992
  Scope3 : Scope  NumInputPorts=3
  Scope4 : Scope  NumInputPorts=6
      settings: ActiveDisplayYMinimum=-20.488040447235107  ActiveDisplayYMaximum=15.403716564178467  DataLoggingVariableName=ScopeData11
  Sum7 : Sum  Inputs=-+
  Terminator : Terminator
  wrap2Pi : Subsystem
  path_moni : Outport
  d/dt_gachiv_e : Outport  Port=2  PortDimensions=3
  wires:
  phi_m/1 -> MATLAB Function2/1(phi)
  para/1 -> Bus Selector1/1, Bus Selector2/1
  Add/1 -> Mux2/1
  Sum7/1 -> Demux1/1
  Mux2/1 -> Minus/1, Gain3/1
  Bus Selector1/1 -> Product2/1  "<K_TRK_GAMMAI>"
  gachiv_m/1 -> Sum7/1, Gain1/1
  Demux/1 -> Add/1, Mux3/1
  Add1/1 -> Mux2/2
  MATLAB Function2/1(gamma_dot_ffw) -> Add/2
  Demux/3 -> Mux2/3
  Gain7/1 -> Scope4/3
  d/dt_gachiv_m/1 -> Minus/2, Gain6/1
  Demux1/2 -> wrap2Pi/1(In1)
  wrap2Pi/1(Out1) -> Mux4/2
  Demux1/3 -> Mux4/3
  Demux1/1 -> Mux4/1, Discrete-Time Integrator/1
  Bus Selector2/1 -> Mux6/1  "<K_TRK_GAMMA>"
  Bus Selector2/2 -> Mux6/2  "<K_TRK_CHI>"
  Bus Selector2/3 -> Mux6/3  "<K_TRK_V>"
  Mux3/1 -> Gain4/1
  Mux7/1 -> Gain8/1
  Minus/1 -> Gain14/1, Gain7/1, Gain9/1, d/dt_gachiv_e/1
  Gain10/1 -> Scope4/4
  Gain14/1 -> Minus2/2, Scope3/2
  Minus2/1 -> Scope3/1
  gachiv_c/1 -> Sum7/2, Gain5/1
  Gain5/1 -> Bus Creator/1, Scope/1
  Gain1/1 -> Bus Creator/2, Scope/2
  Gain2/1 -> Bus Creator/3, Scope/3
  Gain4/1 -> Bus Creator/4, Scope/4
  Gain3/1 -> Bus Creator/6, Scope4/1, Scope/6
  Gain6/1 -> Bus Creator/7, Scope4/2
  Gain9/1 -> Bus Creator/8, Scope4/6, Minus2/1, Scope3/3
  Gain8/1 -> Bus Creator/5, Scope/5
  Bus Creator/1 -> path_moni/1
  Mux6/1 -> Product/2
  Constant2/1 -> Product2/2, Discrete-Time Integrator/2
  Discrete-Time Integrator/1 -> Product2/3
  Product/1 -> Demux/1
  Demux/2 -> Mux7/1, Add1/2
  Constant/1 -> Add1/1
  Product2/1 -> Mux3/2
  Constant1/1 -> Mux7/2
  Mux4/1 -> Gain2/1, Product/1
  Bus Selector2/5 -> Mux1/2  "<K_TRK_V_CLB>"
  Bus Selector2/4 -> Mux1/1  "<K_TRK_GA_CLB>"
  Mux1/1 -> Terminator/1

== system gnc/INDI/Rates to surfaces&brakes/Diff and Filter IMU ==
  note: Use filtered derivative of angular velocities from IMU filter module or filter here
  imu_filter : Inport
  act_m : Inport  Port=2
  rates : Inport  Port=3
  params : Inport  Port=4  OutDataTypeStr=Bus: gnc_parameterBus
  Bus Selector : BusSelector  OutputSignals=imu_filt_ang_acc
  Bus Selector1 : BusSelector  OutputSignals=ang_acc
  Bus Selector2 : BusSelector  OutputSignals=omega,zeta
  Discrete Transfer Fcn : DiscreteTransferFcn  LoadFcn=dspblkCoreblockFVToolHelper(gcbh,'load');  NumeratorSource=Input port  DenominatorSource=Input port  a0EqualsOne=on
      settings: CopyFcn=dspblkCoreblockFVToolHelper(gcbh,'copy');  DeleteFcn=dspblkCoreblockFVToolHelper(gcbh,'close');  ModelCloseFcn=dspblkCoreblockFVToolHelper(gcbh,'close');  PreSaveFcn=dspblkCoreblockFVToolHelper(gcbh,'presave');  PostSaveFcn=dspblkCoreblockFVToolHelper(gcbh,'postsave');  CloseFcn=dspblkCoreblockFVToolHelper(gcbh,'close');  InputPortMap=u0,p1,p3
  MATLAB Function : MATLAB Function  TreatAsAtomicUnit=on
  Scope : Scope  NumInputPorts=2
      settings: ActiveDisplayYMinimum=-7.9407268166542053  ActiveDisplayYMaximum=7.8752565979957581  DataLoggingVariableName=ScopeData24
  Selector : Selector  InputPortWidth=4  IndexOptions=Index vector (dialog)  Indices=1:3  OutputSizes=1
  Subsystem : Subsystem
  Switch : Switch  Criteria=u2 > Threshold  SaturateOnIntegerOverflow=off  InputSameDT=off
  Switch1 : Switch  Criteria=u2 > Threshold  SaturateOnIntegerOverflow=off  InputSameDT=off
  fromRPAS : Subsystem  Commented=on
  act_del : Outport  OutDataTypeStr=single  PortDimensions=3
  d/dt_pqr_m : Outport  Port=2  OutDataTypeStr=single  PortDimensions=3
  wires:
  act_m/1 -> Selector/1
  Selector/1 -> Subsystem/2(act_m), Discrete Transfer Fcn/1
  MATLAB Function/1(num) -> Discrete Transfer Fcn/2
  MATLAB Function/2(den) -> Discrete Transfer Fcn/3
  imu_filter/1 -> Bus Selector2/1, Bus Selector1/1
  rates/1 -> Subsystem/1(rates)
  Switch1/1 -> d/dt_pqr_m/1
  Switch/1 -> act_del/1
  Subsystem/2(act_del) -> Switch/3
  Discrete Transfer Fcn/1 -> Switch/1
  Bus Selector/1 -> Switch/2, Switch1/2  "<imu_filt_ang_acc>"
  Subsystem/1(dt_pqr_m) -> Switch1/3, Scope/1
  Bus Selector1/1 -> Scope/2, Switch1/1  "<ang_acc>"
  params/1 -> Bus Selector/1
  Bus Selector2/1 -> MATLAB Function/1(omega)  "<omega>"
  Bus Selector2/2 -> MATLAB Function/2(zeta)  "<zeta>"

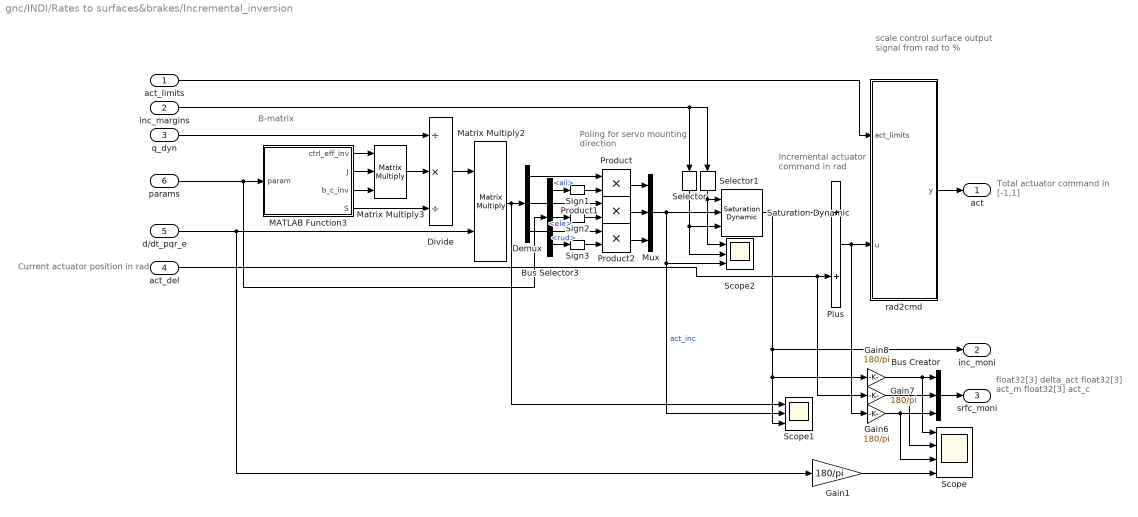
== system gnc/INDI/Rates to surfaces&brakes/Incremental_inversion ==
  note: B-matrix
  note: float32[3] delta_act
      | float32[3] act_m
      | float32[3] act_c
  note: Incremental
      | actuator
      | command
      | in rad
  note: Current actuator position in rad
  note: scale control
      | surface output
      | signal from
      | rad to %
  note: Total actuator
      | command in [-1,1]
  note: Poling for servo
      | mounting direction
  act_limits : Inport
  inc_margins : Inport  Port=2  OutDataTypeStr=single  PortDimensions=[3,2]
  q_dyn : Inport  Port=3
  act_del : Inport  Port=4  OutDataTypeStr=single  PortDimensions=3
  d/dt_pqr_e : Inport  Port=5
  params : Inport  Port=6  OutDataTypeStr=Bus: gnc_parameterBus
  Bus Creator : BusCreator  Inputs=3
  Bus Selector3 : BusSelector  OutputSignals=controlsigns.ail,controlsigns.ele,controlsigns.rud
  Demux : Demux  Outputs=3
  Divide : Product  Inputs=/*/
  Gain{1,6..8} (4 alike) : Gain  Gain=180/pi
  MATLAB Function3 : MATLAB Function  TreatAsAtomicUnit=on
  Matrix Multiply2 : Product  Multiplication=Matrix(*)
  Matrix Multiply3 : Product  Inputs=3  Multiplication=Matrix(*)
  Mux : Mux  Inputs=3
  Plus : Sum
  Product : Product  OutDataTypeStr=single
  Product1 : Product  OutDataTypeStr=single
  Product2 : Product  OutDataTypeStr=single
  Saturation Dynamic : simulink/Discontinuities/Saturation Dynamic  OutMin=[]  OutMax=[]  OutDataTypeStr=Inherit: Same as second input  OutDataType=fixdt(1, 16)  OutScaling=2^-10  DoSatur=off
  Scope : Scope  NumInputPorts=4
      settings: ActiveDisplayYMinimum=-16.44591760635376  ActiveDisplayYMaximum=26.1960129737854
  Scope1 : Scope  NumInputPorts=3
      settings: ActiveDisplayYMinimum=-10.004178524017334  ActiveDisplayYMaximum=9.8660979270935059
  Scope2 : Scope  NumInputPorts=3
      settings: ActiveDisplayYMinimum=-0.59764588236630312  ActiveDisplayYMaximum=0.730759123454152  DataLoggingVariableName=ScopeData21
  Selector : Selector  NumberOfDimensions=2  InputPortWidth=3  IndexOptions=Index vector (dialog),Index vector (dialog)  Indices=1:3,1  OutputSizes=1,1
  Selector1 : Selector  NumberOfDimensions=2  InputPortWidth=3  IndexOptions=Index vector (dialog),Index vector (dialog)  Indices=1:3,2  OutputSizes=1,1
  Sign1 : Signum
  Sign2 : Signum
  Sign3 : Signum
  rad2cmd : MATLAB Function  TreatAsAtomicUnit=on
  act : Outport
  inc_moni : Outport  Port=2
  srfc_moni : Outport  Port=3  OutDataTypeStr=single  PortDimensions=9
  wires:
  Matrix Multiply2/1 -> Scope1/1, Demux/1
  Mux/1 -> Scope1/2, Scope2/3, Saturation Dynamic/2  "act_inc"
  act_del/1 -> Gain7/1, Plus/2
  Plus/1 -> Gain6/1, rad2cmd/2(u)
  Saturation Dynamic/1 -> Gain8/1, Scope1/3, inc_moni/1, Plus/1
  rad2cmd/1(y) -> act/1
  MATLAB Function3/3(b_c_inv) -> Matrix Multiply3/3
  MATLAB Function3/1(ctrl_eff_inv) -> Matrix Multiply3/1
  MATLAB Function3/2(J) -> Matrix Multiply3/2
  d/dt_pqr_e/1 -> Matrix Multiply2/2, Gain1/1
  Matrix Multiply3/1 -> Divide/2
  MATLAB Function3/4(S) -> Divide/3
  Divide/1 -> Matrix Multiply2/1
  Bus Creator/1 -> srfc_moni/1
  Gain1/1 -> Scope/4
  Gain8/1 -> Scope/1, Bus Creator/1
  Gain7/1 -> Bus Creator/2, Scope/2
  Gain6/1 -> Scope/3, Bus Creator/3
  act_limits/1 -> rad2cmd/1(act_limits)
  q_dyn/1 -> Divide/1
  params/1 -> Bus Selector3/1, MATLAB Function3/1(param)
  inc_margins/1 -> Selector/1, Selector1/1
  Selector1/1 -> Scope2/1, Saturation Dynamic/1
  Selector/1 -> Scope2/2, Saturation Dynamic/3
  Demux/2 -> Product1/1
  Bus Selector3/3 -> Sign3/1  "<rud>"
  Bus Selector3/1 -> Sign1/1  "<ail>"
  Demux/1 -> Product/1
  Bus Selector3/2 -> Sign2/1  "<ele>"
  Sign1/1 -> Product/2
  Demux/3 -> Product2/1
  Sign2/1 -> Product1/2
  Sign3/1 -> Product2/2
  Product2/1 -> Mux/3
  Product/1 -> Mux/1
  Product1/1 -> Mux/2

== system gnc/INDI/Rates to surfaces&brakes/Pseudo-control ==
  note: Feedforward
  note: float32 chi_dot_cmd
      | float32 chi_dot_m
      | float32 chi_dot_err
      | float32 chi_ddot_cmd
      | float32[3] pqr_cmd
      | float32[3] pqr_m
      | float32[3] pqr_err
      | float32[3] pqr_dot_cmd
      | float32[3] pqr_dot_m
      | float32[3] pqr_dot_err
  pqr_dot_m : Inport  OutDataTypeStr=single  PortDimensions=3
  rate_m : Inport  Port=2  OutDataTypeStr=single  PortDimensions=3
  rte_c : Inport  Port=3  OutDataTypeStr=single  PortDimensions=3
  param : Inport  Port=4  OutDataTypeStr=Bus: gnc_parameterBus
  Bus Creator : BusCreator  Inputs=10
  Bus Selector : BusSelector  OutputSignals=indi.K_RTE_PSI_DD,indi.K_RTE_P,indi.K_RTE_Q,indi.K_RTE_R
  Constant1 : Constant  Value=0  OutDataTypeStr=single
  Gain{1..5,7..9} (8 alike) : Gain  Gain=180/pi
  Mux10 : Mux  Inputs=3
  Product3 : Product
  Scope : Scope  NumInputPorts=4
      settings: ActiveDisplayYMinimum=-71.076124972607658  ActiveDisplayYMaximum=83.841861334191776  DataLoggingVariableName=ScopeData2
  Scope2 : Scope  NumInputPorts=4
      settings: ActiveDisplayYMinimum=-1266.2567672729492  ActiveDisplayYMaximum=2019.7770919799805  DataLoggingVariableName=ScopeData2
  Sum1 : Sum  Inputs=+-|
  Sum22 : Sum  Inputs=-+|
  d/dt_pqr_e : Outport  OutDataTypeStr=single  PortDimensions=3
  rte_moni : Outport  Port=2  OutDataTypeStr=single  PortDimensions=22
  wires:
  Mux10/1 -> Product3/1  "ail ele rud"
  Sum22/1 -> Gain3/1, Product3/2
  rate_m/1 -> Gain1/1, Sum22/1
  Bus Selector/2 -> Mux10/1  "<K_RTE_P>"
  Bus Selector/3 -> Mux10/2  "<K_RTE_Q>"
  param/1 -> Bus Selector/1
  rte_c/1 -> Sum22/2, Gain2/1
  Bus Selector/4 -> Mux10/3  "<K_RTE_R>"
  Product3/1 -> Gain8/1, Sum1/1, Gain9/1
  Gain3/1 -> Scope/2, Bus Creator/7
  Gain9/1 -> Scope/1
  Gain8/1 -> Scope2/3, Bus Creator/8
  Gain1/1 -> Scope/3, Bus Creator/6
  Bus Selector/1 -> ?  "<K_RTE_PSI_DD>"
  Gain2/1 -> Scope/4, Bus Creator/5
  Sum1/1 -> d/dt_pqr_e/1, Gain5/1
  pqr_dot_m/1 -> Gain4/1, Sum1/2
  Gain4/1 -> Scope2/2, Bus Creator/9
  Gain5/1 -> Bus Creator/10, Scope2/1
  Bus Creator/1 -> rte_moni/1
  Gain7/1 -> Scope2/4
  Constant1/1 -> Bus Creator/2, Bus Creator/3, Bus Creator/4, Bus Creator/1
